simulink model "VehicleWithABS"  (R2014b)
settings: Solver=ode3  StartTime=0.0  StopTime=6  FixedStep=0.01  RelTol=1e-3
settings Model: Creator=树下曼荼罗  LastModifiedBy=树下曼荼罗

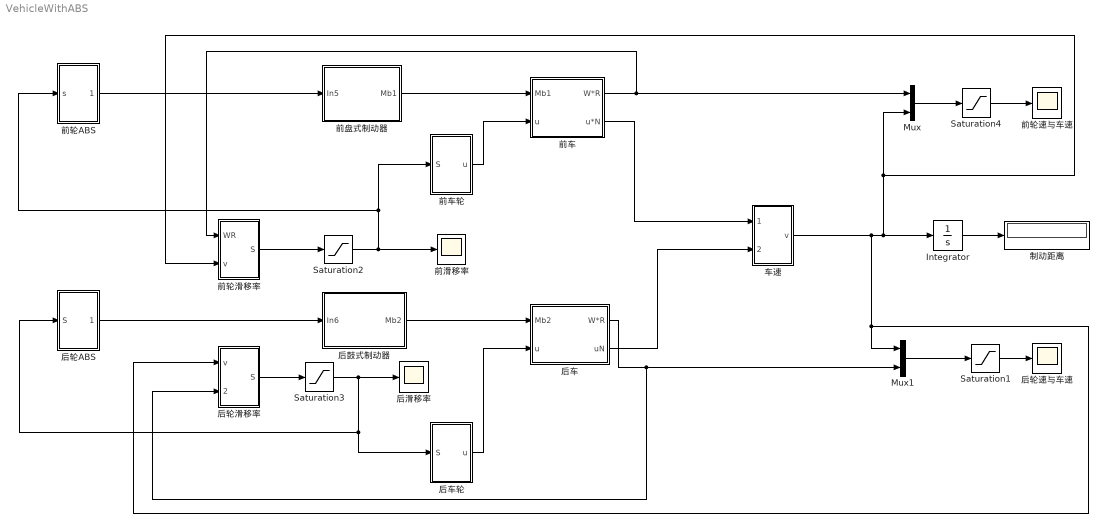
== system VehicleWithABS ==
  Integrator : Integrator
  Mux : Mux  Inputs=2
  Mux1 : Mux  Inputs=2
  Saturation1 : Saturate  UpperLimit=25  LowerLimit=0
  Saturation2 : Saturate  UpperLimit=1  LowerLimit=0
  Saturation3 : Saturate  UpperLimit=1  LowerLimit=0
  Saturation4 : Saturate  UpperLimit=25  LowerLimit=0
  制动距离 : Display
  前滑移率 : Scope
      settings: ShowLegends=on  TimeRange=4  SaveName=ScopeData2  ScrollMode=on
  前盘式制动器 : Subsystem
  前车 : Subsystem
  前车轮 : Subsystem
  前轮ABS : Subsystem
  前轮滑移率 : Subsystem
  前轮速与车速 : Scope
      settings: TickLabels=on  ShowLegends=on  TimeRange=4  YMin=0  YMax=25  ScrollMode=on
  后滑移率 : Scope
      settings: TickLabels=on  ShowLegends=on  SaveName=ScopeData3  ScrollMode=on
  后车 : Subsystem
  后车轮 : Subsystem
  后轮ABS : Subsystem
  后轮滑移率 : Subsystem
  后轮速与车速 : Scope
      settings: ShowLegends=on  TimeRange=4  YMin=-50  YMax=30  ScrollMode=on
  后鼓式制动器 : Subsystem
  车速 : Subsystem
  wires:
  后车轮/1(u) -> 后车/2(u)
  后车/1(W*R) -> 后轮滑移率/2(W*R), Mux1/2
  Integrator/1 -> 制动距离/1
  Mux1/1 -> Saturation1/1
  前盘式制动器/1(Mb1) -> 前车/1(Mb1)
  后鼓式制动器/1(Mb2) -> 后车/1(Mb2)
  前车轮/1(u) -> 前车/2(u)
  前车/1(W*R) -> 前轮滑移率/1(WR), Mux/1
  Mux/1 -> Saturation4/1
  Saturation1/1 -> 后轮速与车速/1
  Saturation2/1 -> 前轮ABS/1(s), 前车轮/1(S), 前滑移率/1
  Saturation3/1 -> 后车轮/1(S), 后轮ABS/1(S), 后滑移率/1
  Saturation4/1 -> 前轮速与车速/1
  车速/1(v) -> Mux1/1, 后轮滑移率/1(v), Mux/2, 前轮滑移率/2(v), Integrator/1
  前车/2(u*N) -> 车速/1(前uN)
  后车/2(uN) -> 车速/2(后uN)
  前轮滑移率/1(S) -> Saturation2/1
  后轮滑移率/1(S) -> Saturation3/1
  前轮ABS/1(Out1) -> 前盘式制动器/1(In5)
  后轮ABS/1(Out1) -> 后鼓式制动器/1(In6)

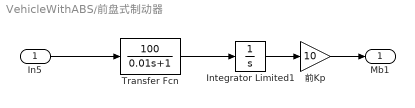
== system VehicleWithABS/前盘式制动器 ==
  In5 : Inport
  Integrator Limited1 : Integrator  UpperSaturationLimit=1  LowerSaturationLimit=0
  Transfer Fcn : TransferFcn  Numerator=[100]  Denominator=[0.01 1]
  前Kp : Gain  Gain=10
  Mb1 : Outport
  wires:
  前Kp/1 -> Mb1/1
  In5/1 -> Transfer Fcn/1
  Transfer Fcn/1 -> Integrator Limited1/1
  Integrator Limited1/1 -> 前Kp/1

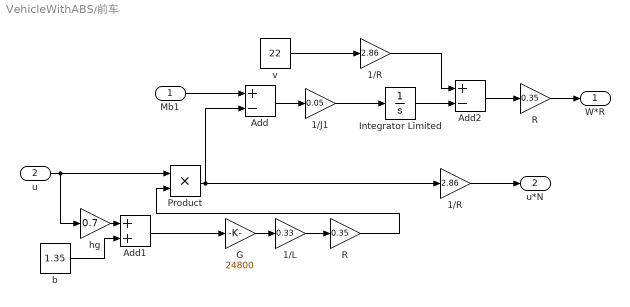
== system VehicleWithABS/前车 ==
  Mb1 : Inport
  u : Inport  Port=2
  1/J1 : Gain  Gain=0.05
  1/L : Gain  Gain=0.33
  1/R : Gain  Gain=2.86
  "1/R " : Gain  Gain=2.86
  Add : Sum  Inputs=+-
  Add1 : Sum
  Add2 : Sum  Inputs=+-
  G : Gain  Gain=24800
  Integrator Limited : Integrator  UpperSaturationLimit=1  LowerSaturationLimit=0
  Product : Product
  R : Gain  Gain=0.35
  "R " : Gain  Gain=0.35
  b : Constant  Value=1.35
  hg : Gain  Gain=0.7
  v : Constant  Value=22
  W*R : Outport
  u*N : Outport  Port=2
  wires:
  R/1 -> W*R/1
  Add1/1 -> G/1
  Add/1 -> 1/J1/1
  Product/1 -> Add/2, "1/R "/1
  b/1 -> Add1/2
  u/1 -> Product/1, hg/1
  1/L/1 -> "R "/1
  G/1 -> 1/L/1
  hg/1 -> Add1/1
  Mb1/1 -> Add/1
  "R "/1 -> Product/2
  1/J1/1 -> Integrator Limited/1
  v/1 -> 1/R/1
  1/R/1 -> Add2/1
  Integrator Limited/1 -> Add2/2
  Add2/1 -> R/1
  "1/R "/1 -> u*N/1

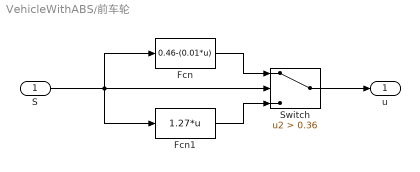
== system VehicleWithABS/前车轮 ==
  S : Inport
  Fcn : Fcn  Expr=0.46-(0.01*u)
  Fcn1 : Fcn  Expr=1.27*u
  Switch : Switch  Criteria=u2 > Threshold  Threshold=0.36
  u : Outport
  wires:
  S/1 -> Fcn/1, Switch/2, Fcn1/1
  Fcn/1 -> Switch/1
  Fcn1/1 -> Switch/3
  Switch/1 -> u/1

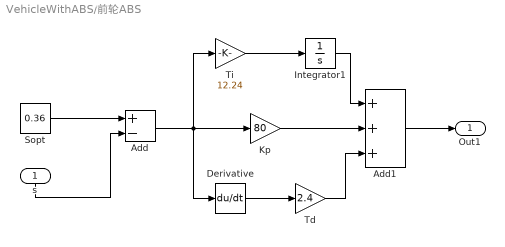
== system VehicleWithABS/前轮ABS ==
  s : Inport
  Add : Sum  Inputs=+-
  Add1 : Sum  Inputs=+++
  Derivative : Derivative
  Integrator1 : Integrator
  Kp : Gain  Gain=80
  Sopt : Constant  Value=0.36
  Td : Gain  Gain=2.4
  Ti : Gain  Gain=12.24
  Out1 : Outport
  wires:
  s/1 -> Add/2
  Ti/1 -> Integrator1/1
  Kp/1 -> Add1/2
  Integrator1/1 -> Add1/1
  Add/1 -> Derivative/1, Ti/1, Kp/1
  Sopt/1 -> Add/1
  Add1/1 -> Out1/1
  Derivative/1 -> Td/1
  Td/1 -> Add1/3

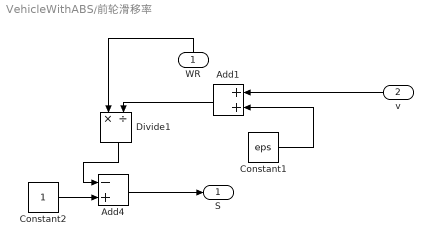
== system VehicleWithABS/前轮滑移率 ==
  WR : Inport
  v : Inport  Port=2
  Add1 : Sum
  Add4 : Sum  Inputs=-+
  Constant1 : Constant  Value=eps
  Constant2 : Constant
  Divide1 : Product  Inputs=*/
  S : Outport
  wires:
  Constant2/1 -> Add4/2
  Divide1/1 -> Add4/1
  Add4/1 -> S/1
  WR/1 -> Divide1/1
  v/1 -> Add1/1
  Add1/1 -> Divide1/2
  Constant1/1 -> Add1/2

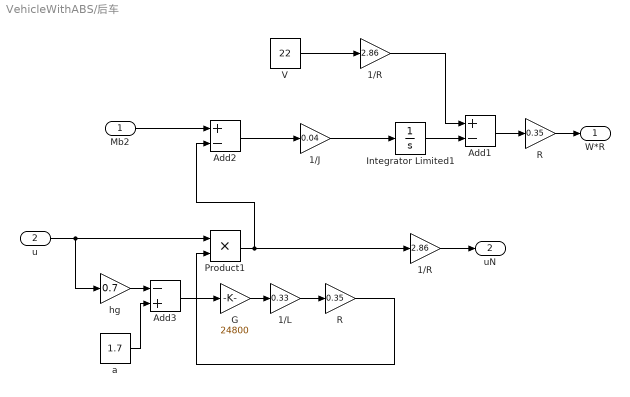
== system VehicleWithABS/后车 ==
  Mb2 : Inport
  u : Inport  Port=2
  1/J : Gain  Gain=0.04
  1/L : Gain  Gain=0.33
  1/R : Gain  Gain=2.86
  "1/R " : Gain  Gain=2.86
  Add1 : Sum  Inputs=+-
  Add2 : Sum  Inputs=+-
  Add3 : Sum  Inputs=-+
  G : Gain  Gain=24800
  Integrator Limited1 : Integrator  UpperSaturationLimit=1  LowerSaturationLimit=0
  Product1 : Product
  R : Gain  Gain=0.35
  "R " : Gain  Gain=0.35
  V : Constant  Value=22
  a : Constant  Value=1.7
  hg : Gain  Gain=0.7
  W*R : Outport
  uN : Outport  Port=2
  wires:
  Product1/1 -> "1/R "/1, Add2/2
  Mb2/1 -> Add2/1
  R/1 -> W*R/1
  G/1 -> 1/L/1
  Add2/1 -> 1/J/1
  1/J/1 -> Integrator Limited1/1
  u/1 -> hg/1, Product1/1
  hg/1 -> Add3/1
  Add3/1 -> G/1
  1/L/1 -> "R "/1
  a/1 -> Add3/2
  "R "/1 -> Product1/2
  V/1 -> 1/R/1
  1/R/1 -> Add1/1
  Integrator Limited1/1 -> Add1/2
  Add1/1 -> R/1
  "1/R "/1 -> uN/1

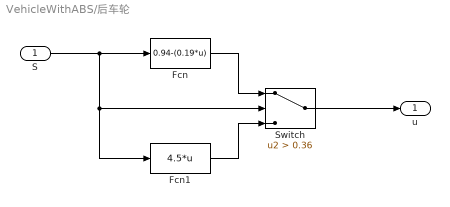
== system VehicleWithABS/后车轮 ==
  S : Inport
  Fcn : Fcn  Expr=0.94-(0.19*u)
  Fcn1 : Fcn  Expr=4.5*u
  Switch : Switch  Criteria=u2 > Threshold  Threshold=0.36
  u : Outport
  wires:
  S/1 -> Switch/2, Fcn1/1, Fcn/1
  Fcn/1 -> Switch/1
  Fcn1/1 -> Switch/3
  Switch/1 -> u/1

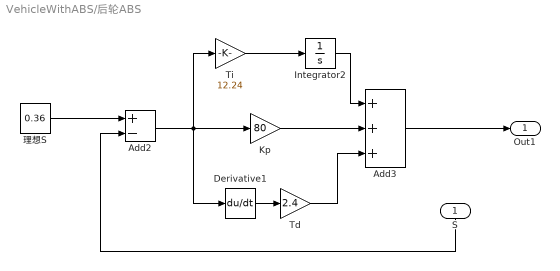
== system VehicleWithABS/后轮ABS ==
  S : Inport
  Add2 : Sum  Inputs=+-
  Add3 : Sum  Inputs=+++
  Derivative1 : Derivative
  Integrator2 : Integrator
  Kp : Gain  Gain=80
  Td : Gain  Gain=2.4
  Ti : Gain  Gain=12.24
  理想S : Constant  Value=0.36
  Out1 : Outport
  wires:
  S/1 -> Add2/2
  Add3/1 -> Out1/1
  Kp/1 -> Add3/2
  Integrator2/1 -> Add3/1
  Ti/1 -> Integrator2/1
  Add2/1 -> Derivative1/1, Kp/1, Ti/1
  Derivative1/1 -> Td/1
  理想S/1 -> Add2/1
  Td/1 -> Add3/3

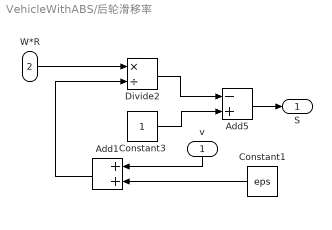
== system VehicleWithABS/后轮滑移率 ==
  v : Inport
  W*R : Inport  Port=2
  Add1 : Sum
  Add5 : Sum  Inputs=-+
  Constant1 : Constant  Value=eps
  Constant3 : Constant
  Divide2 : Product  Inputs=*/
  S : Outport
  wires:
  v/1 -> Add1/1
  Divide2/1 -> Add5/1
  Add5/1 -> S/1
  Constant3/1 -> Add5/2
  Add1/1 -> Divide2/2
  Constant1/1 -> Add1/2
  W*R/1 -> Divide2/1

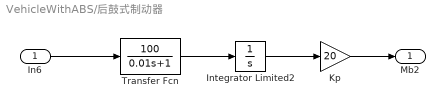
== system VehicleWithABS/后鼓式制动器 ==
  In6 : Inport
  Integrator Limited2 : Integrator  UpperSaturationLimit=1  LowerSaturationLimit=0
  Kp : Gain  Gain=20
  Transfer Fcn : TransferFcn  Numerator=[100]  Denominator=[0.01 1]
  Mb2 : Outport
  wires:
  Kp/1 -> Mb2/1
  Transfer Fcn/1 -> Integrator Limited2/1
  Integrator Limited2/1 -> Kp/1
  In6/1 -> Transfer Fcn/1

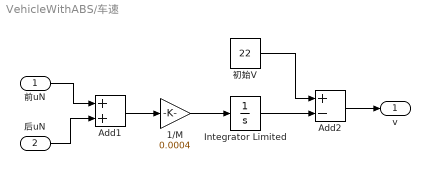
== system VehicleWithABS/车速 ==
  前uN : Inport
  后uN : Inport  Port=2
  1/M : Gain  Gain=0.0004
  Add1 : Sum
  Add2 : Sum  Inputs=+-
  Integrator Limited : Integrator  UpperSaturationLimit=1  LowerSaturationLimit=0
  初始V : Constant  Value=22
  v : Outport
  wires:
  Add2/1 -> v/1
  后uN/1 -> Add1/2
  Add1/1 -> 1/M/1
  Integrator Limited/1 -> Add2/2
  初始V/1 -> Add2/1
  1/M/1 -> Integrator Limited/1
  前uN/1 -> Add1/1
